simulink model "SAME5x_EXpicGUI"  (R2020b)
settings: Solver=FixedStepDiscrete  StartTime=0.0  StopTime=10.0  FixedStep=Ts  RelTol=1e-3  EnableMultiTasking=on
InitFcn:
  | % DC Voltage
  | VDC = 24;
  | 
  | 
  | % Intersective PMW
  | Vmax = VDC/2;
  | Imax = 4;
  | 
  | Ts = 1e-4;
  | 
  | 
  | 
  | 
  | 
  | 
  | % pole paires
  | p = 4;
  | 
  | % QEI
  | lines = 4*1000;
  | eleclines = lines/p;
  | inveleclines = 1/eleclines
  | gainQEIspeed = 2*pi/Ts/lines
  | 
  | 
  | 
  | % Electrical parameters
  | R=0.656; L=0.35e-3; Phif=0.0066;
  | % Mechanical parameters
  | F=1.e-05; J=1e-05; C0 = 0.01;%10;%1;
  | 
  | %% Current control synthesis
  | % Desired Carateristc Equation
  | %  1         2zeta
  | % ---- p^2+ ------- p + 1
  | % wn^2        wn
  | % Overshoot 5%, Trbf x wnbf = 3
  | tauE = L/R;
  | kE = 1/R;
  | trE = 3*tauE;
  | trED = trE;
  | zetaED = 1;
  | trwnE = 5;
  | wnED = trwnE/trED;
  | Pole_elec_desiree = roots([1/wnED^2 2*zetaED/wnED 1]);
  | 
  | % Retour d'etat de la dynamique electrique
  | Ae = [
  |         -R/L 0;
  |         -1 0;
  |     ];
  | 
  | Be = [
  |         1/L;
  |         0;
  |     ];
  | 
  | Kelec = place(Ae,Be,Pole_elec_desiree)
  | Kelec2 = [(2*zetaED*wnED*tauE-1)/kE -tauE*wnED^2/kE]
  | 
  | ... (+50 lines)
undefined symbols (not defined in the file or in its folder): DiscIntNeverNeededParam, gcbh, MCHP_Digital_Input_Callback, MCHP_Digital_Output_Write_Callback, MCHP_Master_Callback, MCHP_OrderInOut, myParam, PA10, PA11, PA12, PA13, pad0, pad1, pad2, pad3, Pin
libraries: simulink x13, MCHP_Blockset x6
(part 3 of 3)

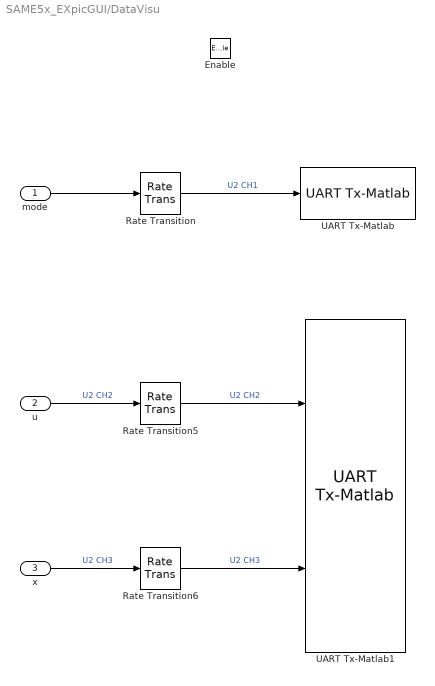
== system SAME5x_EXpicGUI/DataVisu ==
  mode : Inport
  u : Inport  Port=2
  x : Inport  Port=3
  Enable : EnablePort
  Rate Transition : RateTransition
  Rate Transition5 : RateTransition
  Rate Transition6 : RateTransition
  UART Tx-Matlab : MCHP_Blockset/BUS UART/UART Tx-Matlab  UART_REF=2  CHANNELS=[1]  AllOrNothing=off  SampleTime=.1  MCHP_MASTERLINK=SAME5x_EXpicGUI/Microchip Master  MCHP_COMPILED_INFO="CompiledSampleTime= [0.10000000000000000555   0 ];CompiledInportDataTypes=[  5 ];CompiledInportDataWidth=[1];"
      settings: SourceProductName=MPLAB Device Blocks for Simulink
  UART Tx-Matlab1 : MCHP_Blockset/BUS UART/UART Tx-Matlab  UART_REF=2  CHANNELS=[2:3]  AllOrNothing=off  SampleTime=0.0005  MCHP_MASTERLINK=SAME5x_EXpicGUI/Microchip Master  MCHP_COMPILED_INFO="CompiledSampleTime= [0.00050000000000000001041   0 ];CompiledInportDataTypes=[  0   1 ];CompiledInportDataWidth=[1  1];"
      settings: SourceProductName=MPLAB Device Blocks for Simulink
  wires:
  Rate Transition5/1 -> UART Tx-Matlab1/1  "U2 CH2"
  x/1 -> Rate Transition6/1  "U2 CH3"
  Rate Transition6/1 -> UART Tx-Matlab1/2  "U2 CH3"
  u/1 -> Rate Transition5/1  "U2 CH2"
  Rate Transition/1 -> UART Tx-Matlab/1  "U2 CH1"
  mode/1 -> Rate Transition/1

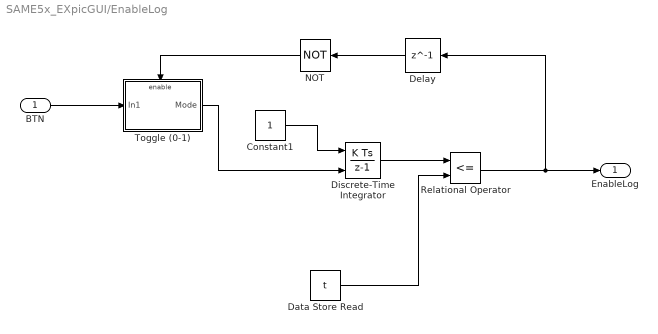
== system SAME5x_EXpicGUI/EnableLog ==
  BTN : Inport
  Constant1 : Constant
  Data Store Read : DataStoreRead  DataStoreName=t  SampleTime=0.1
  Delay : Delay  DelayLength=1
  Discrete-Time Integrator : DiscreteIntegrator  ExternalReset=rising  SampleTime=-1  ICPrevOutput=DiscIntNeverNeededParam  ICPrevScaledInput=DiscIntNeverNeededParam
  NOT : Logic  Operator=NOT  IconShape=distinctive  AllPortsSameDT=off  OutDataTypeStr=boolean
  Relational Operator : RelationalOperator  Operator=<=  OutDataTypeStr=boolean  RndMeth=Simplest
  Toggle (0-1) : Subsystem
  EnableLog : Outport
  wires:
  Data Store Read/1 -> Relational Operator/2
  Discrete-Time Integrator/1 -> Relational Operator/1
  Toggle (0-1)/1(Mode) -> Discrete-Time Integrator/2
  Constant1/1 -> Discrete-Time Integrator/1
  NOT/1 -> Toggle (0-1)/Enable
  Relational Operator/1 -> Delay/1, EnableLog/1
  BTN/1 -> Toggle (0-1)/1(In1)
  Delay/1 -> NOT/1

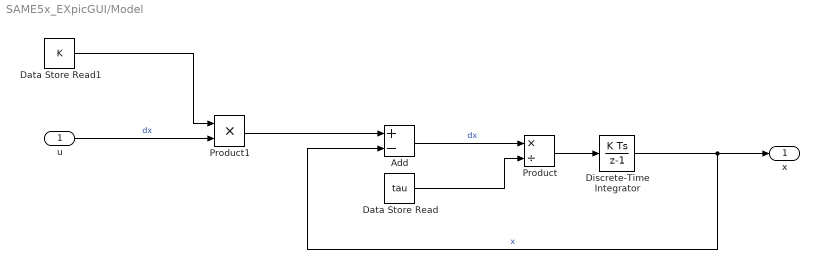
== system SAME5x_EXpicGUI/Model ==
  u : Inport
  Add : Sum  Inputs=+-
  Data Store Read : DataStoreRead  DataStoreName=tau
  Data Store Read1 : DataStoreRead  DataStoreName=K
  Discrete-Time Integrator : DiscreteIntegrator  SampleTime=1e-4  OutDataTypeStr=single  UpperSaturationLimit=100  LowerSaturationLimit=-100  ICPrevOutput=DiscIntNeverNeededParam  ICPrevScaledInput=DiscIntNeverNeededParam
  Product : Product  Inputs=*/
  Product1 : Product
  x : Outport
  wires:
  Add/1 -> Product/1  "dx"
  Discrete-Time Integrator/1 -> x/1, Add/2  "x"
  Product/1 -> Discrete-Time Integrator/1
  Data Store Read/1 -> Product/2
  u/1 -> Product1/2  "dx"
  Product1/1 -> Add/1
  Data Store Read1/1 -> Product1/1

== system SAME5x_EXpicGUI/Modes Serial Terminal  ==
  AND : Logic  IconShape=distinctive  AllPortsSameDT=off  OutDataTypeStr=boolean
  Compare To Zero : simulink/Logic and Bit Operations/Compare To Zero  relop=~=  OutDataTypeStr=boolean
  Space : simulink/Logic and Bit Operations/Compare To Constant  relop=~=  const=32  OutDataTypeStr=boolean
  Subsystem : Subsystem
  UART Rx : MCHP_Blockset/BUS UART/UART Rx  UART_REF=2  Flag_Out=off  Rx_Size_popup=User defined  Rx_Size=1  S_Rx_Size=1  Split=Read all received char  SplitChar=10  OutputDefault_popup=Add one trailing 0  OutputDefault=0  ORDERING=None  SampleTime=.02  MCHP_MASTERLINK=SAME5x_EXpicGUI/Microchip Master  MCHP_COMPILED_INFO="CompiledSampleTime= [0.020000000000000000416   0 ];CompiledInportDataTypes=[    ];CompiledInportDataWidth=[];"
      settings: SourceProductName=MPLAB Device Blocks for Simulink
  modes : Outport
  wires:
  Subsystem/1(modes) -> modes/1
  UART Rx/1 -> Space/1, Subsystem/1(rxBuffer), Compare To Zero/1
  AND/1 -> Subsystem/Enable
  Compare To Zero/1 -> AND/2
  Space/1 -> AND/1

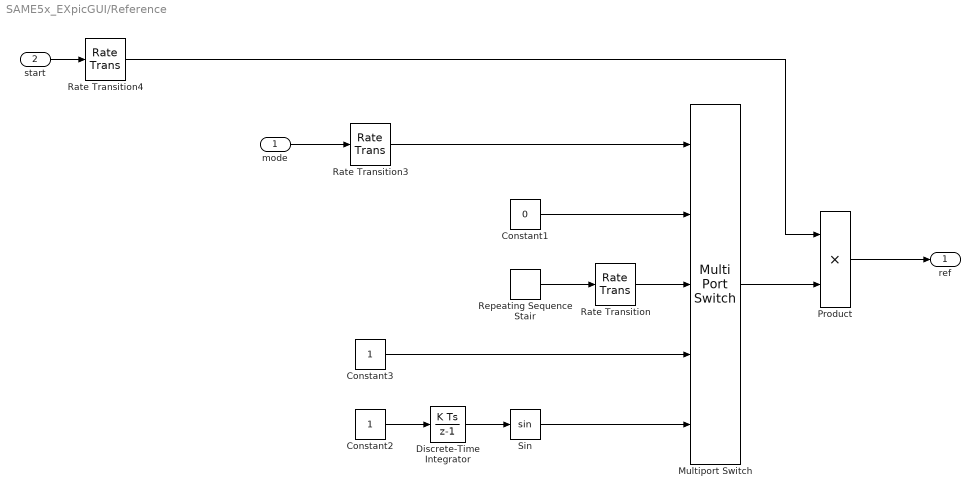
== system SAME5x_EXpicGUI/Reference ==
  mode : Inport
  start : Inport  Port=2
  Constant1 : Constant  Value=0  OutDataTypeStr=single
  Constant2 : Constant  OutDataTypeStr=single
  Constant3 : Constant  OutDataTypeStr=single
  Discrete-Time Integrator : DiscreteIntegrator  SampleTime=-1  ICPrevOutput=DiscIntNeverNeededParam  ICPrevScaledInput=DiscIntNeverNeededParam
  Multiport Switch : MultiPortSwitch  DataPortOrder=Zero-based contiguous  Inputs=4  zeroidx=on
  Product : Product
  Rate Transition : RateTransition
  Rate Transition3 : RateTransition
  Rate Transition4 : RateTransition
  Repeating Sequence Stair : simulink/Sources/Repeating Sequence Stair  OutValues=[0 1].'  tsamp=1  OutMin=[]  OutMax=[]  OutDataTypeStr=double  OutputDataTypeScalingMode=double  OutDataType=fixdt(0,8)  ConRadixGroup=Best Precision: Vector-wise  OutScaling=2^-12
  Sin : Trigonometry
  ref : Outport
  wires:
  mode/1 -> Rate Transition3/1
  Constant2/1 -> Discrete-Time Integrator/1
  Discrete-Time Integrator/1 -> Sin/1
  Constant1/1 -> Multiport Switch/2
  Constant3/1 -> Multiport Switch/4
  Sin/1 -> Multiport Switch/5
  Rate Transition3/1 -> Multiport Switch/1
  Rate Transition4/1 -> Product/1
  Product/1 -> ref/1
  start/1 -> Rate Transition4/1
  Multiport Switch/1 -> Product/2
  Repeating Sequence Stair/1 -> Rate Transition/1
  Rate Transition/1 -> Multiport Switch/3

== system SAME5x_EXpicGUI/EnableLog/Toggle (0-1) ==
  In1 : Inport
  Enable : EnablePort  StatesWhenEnabling=reset
  Bitwise Operator : simulink/Logic and Bit Operations/Bitwise Operator  logicop=AND  UseBitMask=on  BitMask=1  BitMaskRealWorld=Stored Integer
  Change when button is pressed : simulink/Logic and Bit Operations/Detect Decrease  vinit=0.0  OutDataTypeStr=uint8
  Sum : Sum  AccumDataTypeStr=uint16  OutDataTypeStr=uint16
  Unit Delay : UnitDelay  SampleTime=-1  HasFrameUpgradeWarning=on
  Mode : Outport  VectorParamsAs1DForOutWhenUnconnected=off
  wires:
  Change when button is pressed/1 -> Sum/1
  Bitwise Operator/1 -> Mode/1, Unit Delay/1
  Unit Delay/1 -> Sum/2
  Sum/1 -> Bitwise Operator/1
  In1/1 -> Change when button is pressed/1

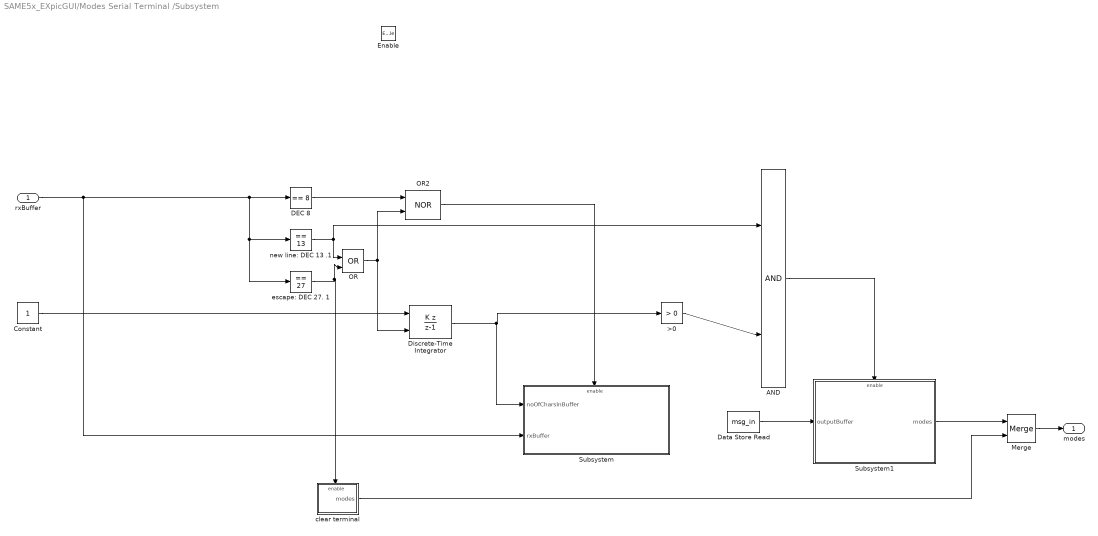
== system SAME5x_EXpicGUI/Modes Serial Terminal /Subsystem ==
  rxBuffer : Inport
  Enable : EnablePort
  >0 : simulink/Logic and Bit Operations/Compare To Constant  relop=>  const=0  OutDataTypeStr=boolean
  AND : Logic  IconShape=distinctive  AllPortsSameDT=off  OutDataTypeStr=boolean
  Constant : Constant  OutDataTypeStr=uint16  SampleTime=-1
  DEC 8 : simulink/Logic and Bit Operations/Compare To Constant  relop===  const=8  OutDataTypeStr=boolean
  Data Store Read : DataStoreRead  DataStoreName=msg_in  SampleTime=.02
  Discrete-Time Integrator : DiscreteIntegrator  IntegratorMethod=Accumulation: Backward Euler  gainval=1  ExternalReset=level  SampleTime=-1  OutDataTypeStr=uint16  ICPrevOutput=DiscIntNeverNeededParam  ICPrevScaledInput=DiscIntNeverNeededParam
  Merge : Merge
  OR : Logic  Operator=OR  IconShape=distinctive  AllPortsSameDT=off  OutDataTypeStr=boolean
  OR2 : Logic  Operator=NOR  IconShape=distinctive  AllPortsSameDT=off  OutDataTypeStr=boolean
  Subsystem : Subsystem
  Subsystem1 : Subsystem
  clear terminal : Subsystem
  escape: DEC 27. 1 : simulink/Logic and Bit Operations/Compare To Constant  relop===  const=27  OutDataTypeStr=boolean
  new line: DEC 13 .1 : simulink/Logic and Bit Operations/Compare To Constant  relop===  const=13  OutDataTypeStr=boolean
  modes : Outport
  wires:
  rxBuffer/1 -> DEC 8/1, new line: DEC 13 .1/1, escape: DEC 27. 1/1, Subsystem/2(rxBuffer)
  >0/1 -> AND/2
  AND/1 -> Subsystem1/Enable
  new line: DEC 13 .1/1 -> OR/1, AND/1
  escape: DEC 27. 1/1 -> clear terminal/Enable, OR/2
  OR/1 -> Discrete-Time Integrator/2, OR2/2
  DEC 8/1 -> OR2/1
  OR2/1 -> Subsystem/Enable
  Constant/1 -> Discrete-Time Integrator/1
  Discrete-Time Integrator/1 -> Subsystem/1(noOfCharsInBuffer), >0/1
  Data Store Read/1 -> Subsystem1/1(outputBuffer)
  Merge/1 -> modes/1
  Subsystem1/1(modes) -> Merge/1
  clear terminal/1(modes) -> Merge/2

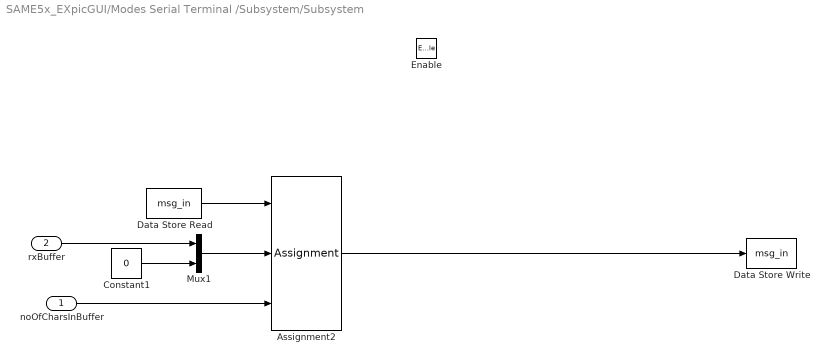
== system SAME5x_EXpicGUI/Modes Serial Terminal /Subsystem/Subsystem ==
  noOfCharsInBuffer : Inport
  rxBuffer : Inport  Port=2
  Enable : EnablePort
  Assignment2 : Assignment  DiagnosticForDimensions=Warning  IndexOptions=Starting index (port)  Indices=1  OutputSizes=1
  Constant1 : Constant  Value=0  OutDataTypeStr=Inherit: Inherit via back propagation
  Data Store Read : DataStoreRead  DataStoreName=msg_in
  Data Store Write : DataStoreWrite  DataStoreName=msg_in
  Mux1 : Mux  Inputs=2
  wires:
  rxBuffer/1 -> Mux1/1
  noOfCharsInBuffer/1 -> Assignment2/3
  Data Store Read/1 -> Assignment2/1
  Mux1/1 -> Assignment2/2
  Constant1/1 -> Mux1/2
  Assignment2/1 -> Data Store Write/1

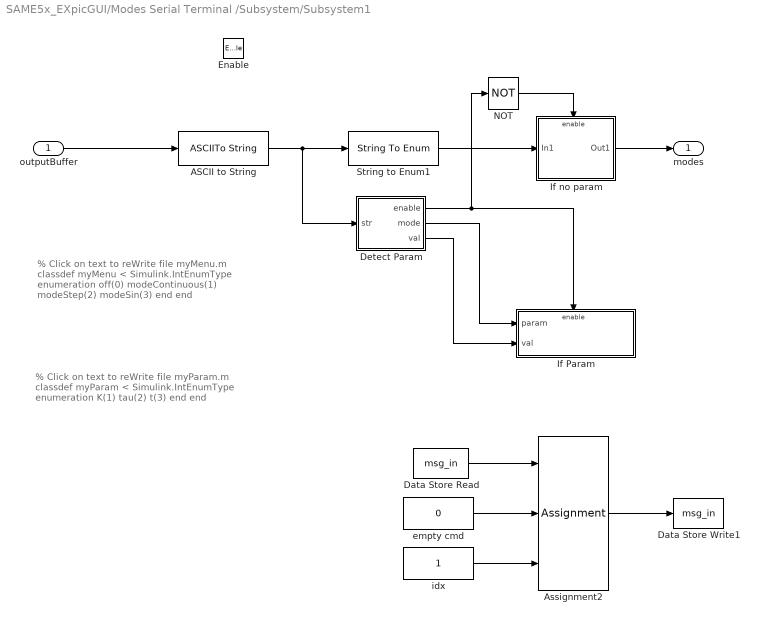
== system SAME5x_EXpicGUI/Modes Serial Terminal /Subsystem/Subsystem1 ==
  note: % Click on text to reWrite file myParam.m
      | classdef myParam < Simulink.IntEnumType
      | enumeration
      | 	K(1)
      | 	tau(2)
      | 	t(3)
      |     end
      | end
  note: % Click on text to reWrite file myMenu.m
      | classdef myMenu < Simulink.IntEnumType
      | enumeration
      | 	off(0)
      | 	modeContinuous(1)
      | 	modeStep(2)
      | 	modeSin(3)
      |     end
      | end
  outputBuffer : Inport
  Enable : EnablePort
  ASCII to String : ASCIIToString
  Assignment2 : Assignment  DiagnosticForDimensions=Warning  IndexOptions=Starting index (port)  Indices=1  OutputSizes=1
  Data Store Read : DataStoreRead  DataStoreName=msg_in
  Data Store Write1 : DataStoreWrite  DataStoreName=msg_in
  "Detect Param " : Subsystem
  If Param : Subsystem
  If no param : Subsystem
  NOT : Logic  Operator=NOT  IconShape=distinctive  AllPortsSameDT=off  OutDataTypeStr=boolean
  String to Enum1 : StringToEnum  OutDataTypeStr=Enum: myMenu
  empty cmd : Constant  Value=0  OutDataTypeStr=uint8
  idx : Constant  OutDataTypeStr=uint8
  modes : Outport
  wires:
  ASCII to String/1 -> "Detect Param "/1(str), String to Enum1/1
  outputBuffer/1 -> ASCII to String/1
  Data Store Read/1 -> Assignment2/1
  Assignment2/1 -> Data Store Write1/1
  empty cmd/1 -> Assignment2/2
  idx/1 -> Assignment2/3
  "Detect Param "/3(val) -> If Param/2(val)
  "Detect Param "/2(mode) -> If Param/1(param)
  "Detect Param "/1(enable) -> NOT/1, If Param/Enable
  String to Enum1/1 -> If no param/1(In1)
  If no param/1(Out1) -> modes/1
  NOT/1 -> If no param/Enable

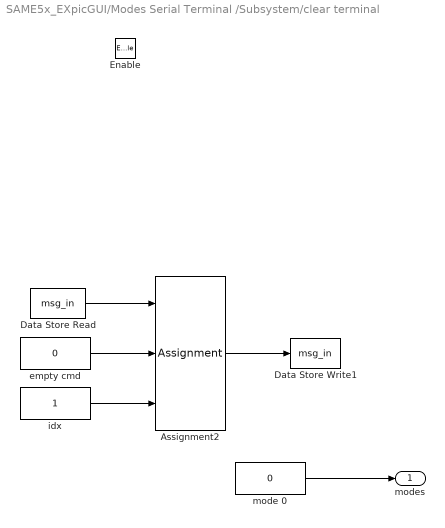
== system SAME5x_EXpicGUI/Modes Serial Terminal /Subsystem/clear terminal ==
  Enable : EnablePort
  Assignment2 : Assignment  DiagnosticForDimensions=Warning  IndexOptions=Starting index (port)  Indices=1  OutputSizes=1
  Data Store Read : DataStoreRead  DataStoreName=msg_in
  Data Store Write1 : DataStoreWrite  DataStoreName=msg_in
  empty cmd : Constant  Value=0  OutDataTypeStr=uint8
  idx : Constant  OutDataTypeStr=uint8
  mode 0 : Constant  Value=0  OutDataTypeStr=uint16
  modes : Outport
  wires:
  empty cmd/1 -> Assignment2/2
  idx/1 -> Assignment2/3
  Data Store Read/1 -> Assignment2/1
  Assignment2/1 -> Data Store Write1/1
  mode 0/1 -> modes/1

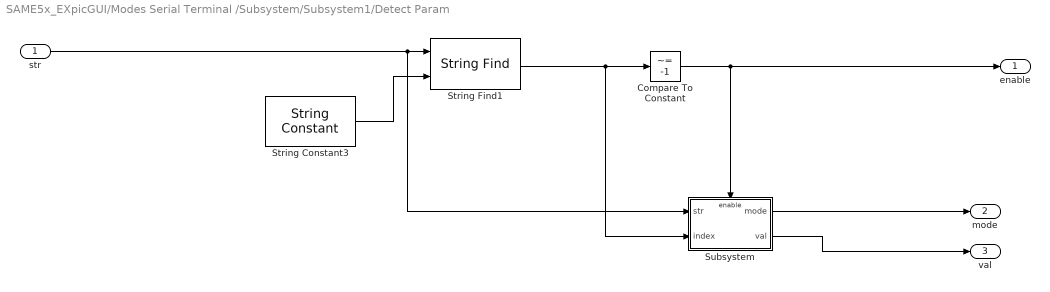
== system SAME5x_EXpicGUI/Modes Serial Terminal /Subsystem/Subsystem1/Detect Param  ==
  str : Inport
  Compare To Constant : simulink/Logic and Bit Operations/Compare To Constant  relop=~=  const=-1  OutDataTypeStr=boolean
  String Constant3 : StringConstant  String="\"=\""
  String Find1 : StringFind
  Subsystem : Subsystem
  enable : Outport
  mode : Outport  Port=2
  val : Outport  Port=3
  wires:
  str/1 -> Subsystem/1(str), String Find1/1
  String Constant3/1 -> String Find1/2
  String Find1/1 -> Subsystem/2(index), Compare To Constant/1
  Subsystem/1(mode) -> mode/1
  Subsystem/2(val) -> val/1
  Compare To Constant/1 -> enable/1, Subsystem/Enable

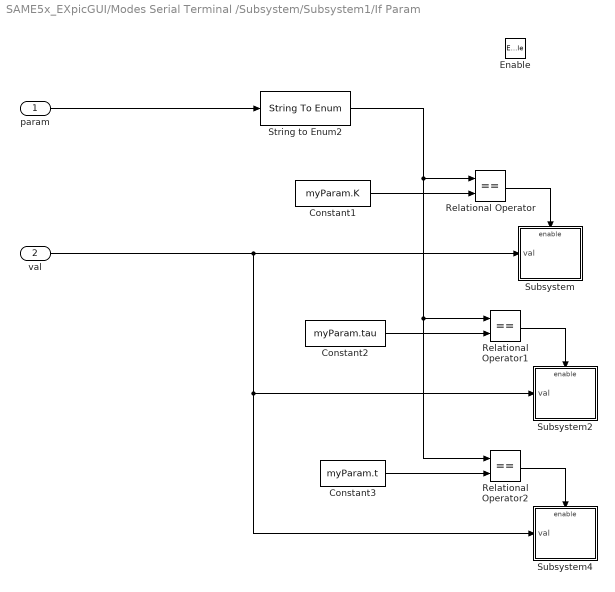
== system SAME5x_EXpicGUI/Modes Serial Terminal /Subsystem/Subsystem1/If Param ==
  param : Inport
  val : Inport  Port=2
  Enable : EnablePort
  Constant1 : Constant  Value=myParam.K  OutDataTypeStr=Enum: myParam
  Constant2 : Constant  Value=myParam.tau  OutDataTypeStr=Enum: myParam
  Constant3 : Constant  Value=myParam.t  OutDataTypeStr=Enum: myParam
  Relational Operator : RelationalOperator  Operator===  OutDataTypeStr=boolean  RndMeth=Simplest
  Relational Operator1 : RelationalOperator  Operator===  OutDataTypeStr=boolean  RndMeth=Simplest
  Relational Operator2 : RelationalOperator  Operator===  OutDataTypeStr=boolean  RndMeth=Simplest
  String to Enum2 : StringToEnum  OutDataTypeStr=Enum: myParam
  Subsystem : Subsystem
  Subsystem2 : Subsystem
  Subsystem4 : Subsystem
  wires:
  String to Enum2/1 -> Relational Operator2/1, Relational Operator1/1, Relational Operator/1
  Relational Operator/1 -> Subsystem/Enable
  Constant1/1 -> Relational Operator/2
  val/1 -> Subsystem4/1(val), Subsystem2/1(val), Subsystem/1(val)
  Relational Operator2/1 -> Subsystem4/Enable
  Relational Operator1/1 -> Subsystem2/Enable
  Constant3/1 -> Relational Operator2/2
  param/1 -> String to Enum2/1
  Constant2/1 -> Relational Operator1/2

== system SAME5x_EXpicGUI/Modes Serial Terminal /Subsystem/Subsystem1/If no param ==
  In1 : Inport
  Enable : EnablePort
  Data Type Conversion : DataTypeConversion  OutDataTypeStr=uint16
  Out1 : Outport
  wires:
  In1/1 -> Data Type Conversion/1
  Data Type Conversion/1 -> Out1/1

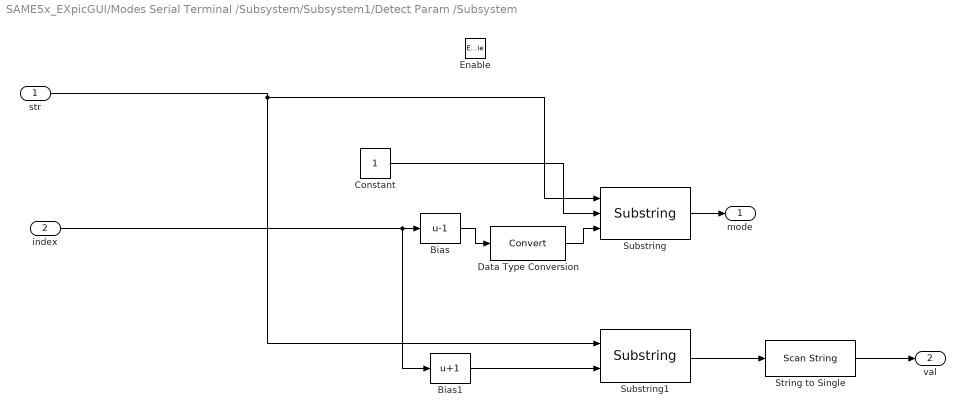
== system SAME5x_EXpicGUI/Modes Serial Terminal /Subsystem/Subsystem1/Detect Param /Subsystem ==
  str : Inport
  index : Inport  Port=2
  Enable : EnablePort
  Bias : Bias  Bias=-1
  Bias1 : Bias  Bias=1
  Constant : Constant  OutDataTypeStr=Inherit: Inherit via back propagation
  Data Type Conversion : DataTypeConversion
  String to Single : ScanString  Format="\"%f\""
  Substring : Substring
  Substring1 : Substring  StringFromIdxToEnd=on
  mode : Outport
  val : Outport  Port=2
  wires:
  Substring1/1 -> String to Single/1
  Constant/1 -> Substring/2
  Substring/1 -> mode/1
  str/1 -> Substring1/1, Substring/1
  Bias1/1 -> Substring1/2
  Data Type Conversion/1 -> Substring/3
  Bias/1 -> Data Type Conversion/1
  index/1 -> Bias1/1, Bias/1
  String to Single/1 -> val/1

== system SAME5x_EXpicGUI/Modes Serial Terminal /Subsystem/Subsystem1/If Param/Subsystem ==
  val : Inport
  Enable : EnablePort
  Data Store Write : DataStoreWrite  DataStoreName=K
  Data Type Conversion : DataTypeConversion  OutDataTypeStr=single
  wires:
  val/1 -> Data Type Conversion/1
  Data Type Conversion/1 -> Data Store Write/1

== system SAME5x_EXpicGUI/Modes Serial Terminal /Subsystem/Subsystem1/If Param/Subsystem2 ==
  val : Inport
  Enable : EnablePort
  Data Store Write : DataStoreWrite  DataStoreName=tau
  Data Type Conversion : DataTypeConversion  OutDataTypeStr=single
  wires:
  Data Type Conversion/1 -> Data Store Write/1
  val/1 -> Data Type Conversion/1

== system SAME5x_EXpicGUI/Modes Serial Terminal /Subsystem/Subsystem1/If Param/Subsystem4 ==
  val : Inport
  Enable : EnablePort
  Data Store Write : DataStoreWrite  DataStoreName=t
  Data Type Conversion : DataTypeConversion
  wires:
  val/1 -> Data Type Conversion/1
  Data Type Conversion/1 -> Data Store Write/1
